simulink model "experimental_1dof"  (R2021a)
settings: Solver=FixedStepAuto  StartTime=0.0  StopTime=250  FixedStep=0.001  RelTol=1e-3
libraries: aerolibatmos2 x1, simulink x1
settings Model: Creator=ctvnu  LastModifiedBy=ctvnu

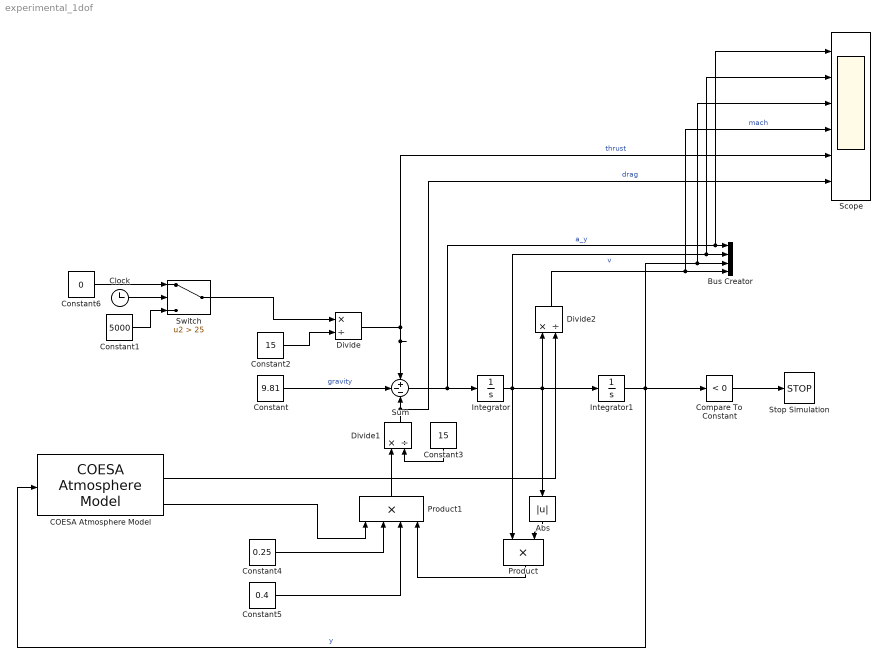
== system experimental_1dof ==
  Abs : Abs
  Bus Creator : BusCreator  Inputs=4
  COESA Atmosphere Model : aerolibatmos2/COESA Atmosphere Model  units=Metric (MKS)  spec=1976 COESA-extended U.S. Standard Atmosphere  model=Profile  profile_var=High temperature  profile_percent=1%  profile_alt=5 km (16404 ft)  envelope_var=High temperature  envelope_percent=1%  action=Warning
  Clock : Clock
  Compare To Constant : simulink/Logic and Bit Operations/Compare To Constant  relop=<  const=0  OutDataTypeStr=boolean
  Constant : Constant  Value=9.81
  Constant1 : Constant  Value=5000
  Constant2 : Constant  Value=15
  Constant3 : Constant  Value=15
  Constant4 : Constant  Value=0.25
  Constant5 : Constant  Value=0.4
  Constant6 : Constant  Value=0
  Divide : Product  Inputs=*/
  Divide1 : Product  Inputs=*/
  Divide2 : Product  Inputs=*/
  Integrator : Integrator
  Integrator1 : Integrator
  Product : Product
  Product1 : Product  Inputs=4
  Scope : Scope  NumInputPorts=6
  Stop Simulation : Stop
  Sum : Sum  Inputs=+--
  Switch : Switch  Criteria=u2 > Threshold  Threshold=25
  wires:
  Sum/1 -> Scope/1, Bus Creator/1, Integrator/1  "a_y"
  Constant/1 -> Sum/2  "gravity"
  Divide/1 -> Scope/5, Sum/1  "thrust"
  Abs/1 -> Product/2
  Integrator/1 -> Bus Creator/2, Scope/2, Divide2/1, Abs/1, Integrator1/1, Product/1  "v"
  Constant1/1 -> Switch/3
  Constant2/1 -> Divide/2
  COESA Atmosphere Model/4 -> Product1/1
  Product1/1 -> Divide1/1
  Constant4/1 -> Product1/2
  Constant5/1 -> Product1/3
  Product/1 -> Product1/4
  Integrator1/1 -> Bus Creator/3, Scope/3, COESA Atmosphere Model/1, Compare To Constant/1  "y"
  Constant6/1 -> Switch/1
  Clock/1 -> Switch/2
  Switch/1 -> Divide/1
  Divide1/1 -> Scope/6, Sum/3  "drag"
  Constant3/1 -> Divide1/2
  Compare To Constant/1 -> Stop Simulation/1
  COESA Atmosphere Model/2 -> Divide2/2
  Divide2/1 -> Scope/4, Bus Creator/4  "mach"
